simulink model "FlightGearIntegration"  (R2022b)
settings: Solver=VariableStepAuto  StartTime=0.0  StopTime=5  RelTol=1e-3
undefined symbols (not defined in the file): Pitch, Roll, Thrust, YawRate
libraries: aerolibfltsims x1, uavalgslib x1, aerolibanimutils x1
settings Model: Creator=skjet  LastModifiedBy=skjet
settings OptimizationCC: BlockReduction=off  DefaultParameterBehavior=Inlined  BufferReuse=off

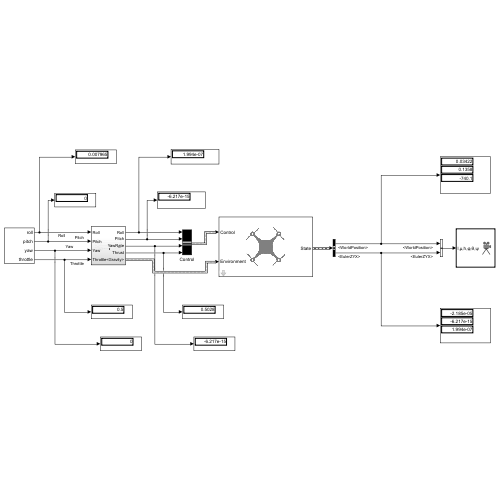
[thumbnail: Simulink's stored preview of the top-level diagram]
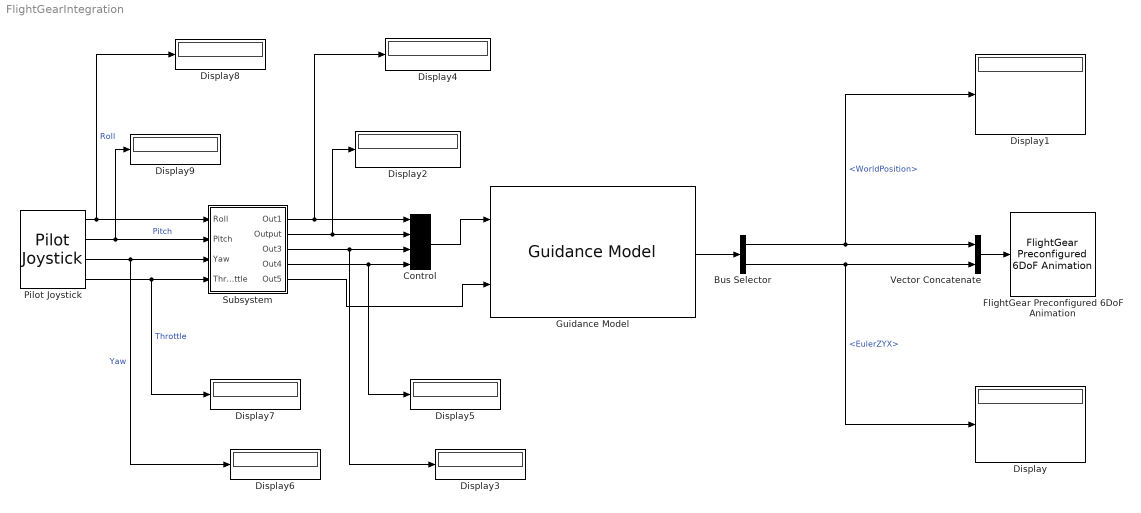
== system FlightGearIntegration ==
  Bus Selector : BusSelector  OutputSignals=WorldPosition,EulerZYX
  Control : BusCreator  Inputs=Roll,Pitch,YawRate,Thrust  OutDataTypeStr=Bus: MultirotorGuidanceControlBus  NonVirtualBus=on
  Display{,1..9} (10 alike) : Display
  FlightGear Preconfigured 6DoF Animation : aerolibfltsims/FlightGear Preconfigured 6DoF Animation  xFlightGearVersion=v2019.1  DestinationIpAddress=127.0.0.1  DestinationPort=5502  SampleTime=1/30  packetVersion=24
  Guidance Model : uavalgslib/Guidance Model  ModelType=MultirotorGuidance  SpecifiedDataType=double  SimulateUsing=Interpreted execution  InitialWorldPositionMultirotor=[0; 0; 0]  InitialWorldVelocityMultirotor=[0; 0; 0]  InitialEulerZYXMultirotor=[0; 0; 0]  InitialBodyAngularRateRPYMultirotor=[0; 0; 0]  InitialThrustMultirotor=0  InitialNorthFixedWing=0  InitialEastFixedWing=0  InitialHeightFixedWing=0  InitialAirSpeedFixedWing=0  InitialHeadingAngleFixedWing=0  InitialFlightPathAngleFixedWing=0  InitialRollAngleFixedWing=0  InitialRollAngleRateFixedWing=0  PDRollMultirotor=[3402.97,116.67]  PDPitchMultirotor=[3402.97, 116.67]  PYawRateMultirotor=1950  PThrustMultirotor=3900  MassMultirotor=0.1  PHeightFixedWing=3.9  PHeadingAngleFixedWing=3.9  PFlightPathAngleFixedWing=39  PDRollFixedWing=[3402.97, 116.67]  PAirSpeedFixedWing=1  FlightPathAngleLimitsFixedWing=[-pi/2, pi/2]  StateBusName='MultirotorGuidanceStateBus'  ControlBusName='MultirotorGuidanceControlBus'  EnvironmentBusName='MultirotorGuidanceEnvironmentBus'  DataType=double
  Pilot Joystick : aerolibanimutils/Pilot Joystick  JoystickID=Joystick1  OutputConfiguration=FourAxis  SampleTime=1/30
  Subsystem : Subsystem
  Vector Concatenate : Concatenate
  wires:
  Pilot Joystick/1 -> Display8/1, Subsystem/1(Roll)  "Roll"
  Pilot Joystick/2 -> Display9/1, Subsystem/2(Pitch)  "Pitch"
  Pilot Joystick/3 -> Display6/1, Subsystem/3(Yaw)  "Yaw"
  Pilot Joystick/4 -> Display7/1, Subsystem/4(Throttle)  "Throttle"
  Guidance Model/1 -> Bus Selector/1
  Bus Selector/1 -> Display1/1, Vector Concatenate/1  "<WorldPosition>"
  Bus Selector/2 -> Display/1, Vector Concatenate/2  "<EulerZYX>"
  Vector Concatenate/1 -> FlightGear Preconfigured 6DoF Animation/1
  Subsystem/5(Out5) -> Guidance Model/2
  Control/1 -> Guidance Model/1
  Subsystem/4(Out4) -> Display5/1, Control/4
  Subsystem/3(Out3) -> Control/3, Display3/1
  Subsystem/2(Output) -> Display2/1, Control/2
  Subsystem/1(Out1) -> Display4/1, Control/1

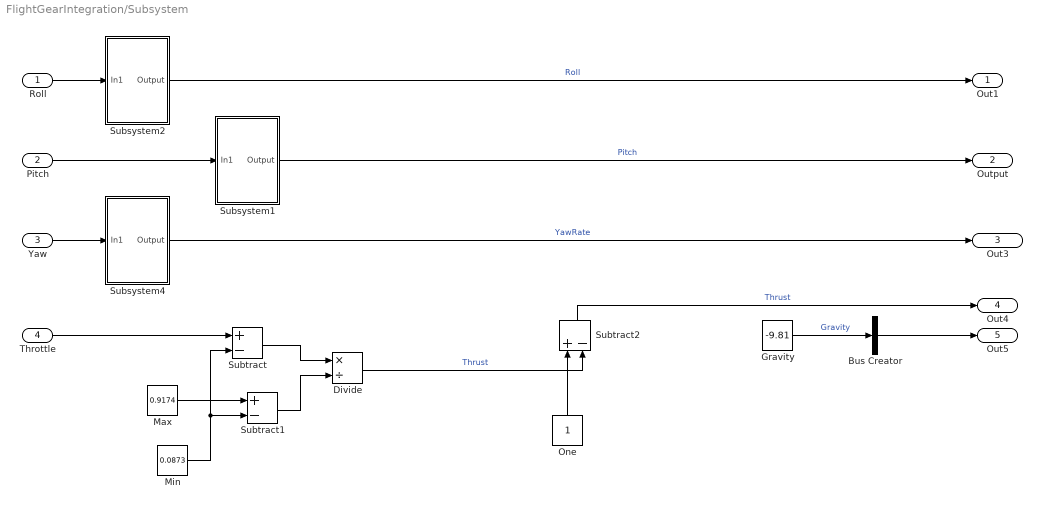
== system FlightGearIntegration/Subsystem ==
  Roll : Inport
  Pitch : Inport  Port=2
  Yaw : Inport  Port=3
  Throttle : Inport  Port=4
  Bus Creator : BusCreator  Inputs=Gravity  OutDataTypeStr=Bus: MultirotorGuidanceEnvironmentBus  NonVirtualBus=on
  Divide : Product  Inputs=*/
  Gravity : Constant  Value=-9.81
  Max : Constant  Value=0.9174
  Min : Constant  Value=0.0873
  One : Constant  OutDataTypeStr=Inherit: Inherit via back propagation
  Subsystem1 : Subsystem
  Subsystem2 : Subsystem
  Subsystem4 : Subsystem
  Subtract : Sum  Inputs=+-
  Subtract1 : Sum  Inputs=+-
  Subtract2 : Sum  Inputs=+-
  Out1 : Outport
  Output : Outport  Port=2
  Out3 : Outport  Port=3
  Out4 : Outport  Port=4
  Out5 : Outport  Port=5
  wires:
  Gravity/1 -> Bus Creator/1  "Gravity"
  Subsystem2/1(Output) -> Out1/1  "Roll"
  Subsystem4/1(Output) -> Out3/1  "YawRate"
  Bus Creator/1 -> Out5/1
  Subsystem1/1(Output) -> Output/1  "Pitch"
  Roll/1 -> Subsystem2/1(In1)
  Yaw/1 -> Subsystem4/1(In1)
  Pitch/1 -> Subsystem1/1(In1)
  Subtract1/1 -> Divide/2
  Min/1 -> Subtract/2, Subtract1/2
  Max/1 -> Subtract1/1
  Subtract/1 -> Divide/1
  Throttle/1 -> Subtract/1
  Divide/1 -> Subtract2/2  "Thrust"
  One/1 -> Subtract2/1
  Subtract2/1 -> Out4/1  "Thrust"

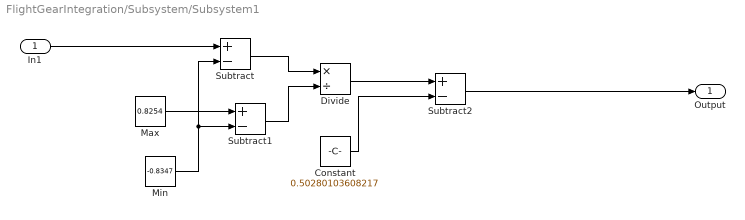
== system FlightGearIntegration/Subsystem/Subsystem1 ==
  In1 : Inport
  Constant : Constant  Value=0.50280103608217
  Divide : Product  Inputs=*/
  Max : Constant  Value=0.8254
  Min : Constant  Value=-0.8347
  Subtract : Sum  Inputs=+-
  Subtract1 : Sum  Inputs=+-
  Subtract2 : Sum  Inputs=+-
  Output : Outport
  wires:
  Divide/1 -> Subtract2/1
  Max/1 -> Subtract1/1
  In1/1 -> Subtract/1
  Min/1 -> Subtract/2, Subtract1/2
  Subtract/1 -> Divide/1
  Subtract1/1 -> Divide/2
  Subtract2/1 -> Output/1
  Constant/1 -> Subtract2/2

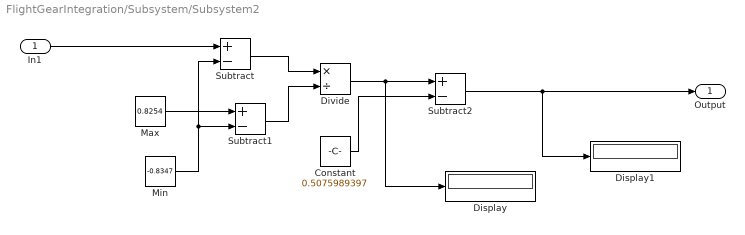
== system FlightGearIntegration/Subsystem/Subsystem2 ==
  In1 : Inport
  Constant : Constant  Value=0.5075989397
  Display : Display
  Display1 : Display
  Divide : Product  Inputs=*/
  Max : Constant  Value=0.8254
  Min : Constant  Value=-0.8347
  Subtract : Sum  Inputs=+-
  Subtract1 : Sum  Inputs=+-
  Subtract2 : Sum  Inputs=+-
  Output : Outport
  wires:
  Divide/1 -> Display/1, Subtract2/1
  Max/1 -> Subtract1/1
  In1/1 -> Subtract/1
  Min/1 -> Subtract/2, Subtract1/2
  Subtract/1 -> Divide/1
  Subtract1/1 -> Divide/2
  Subtract2/1 -> Display1/1, Output/1
  Constant/1 -> Subtract2/2

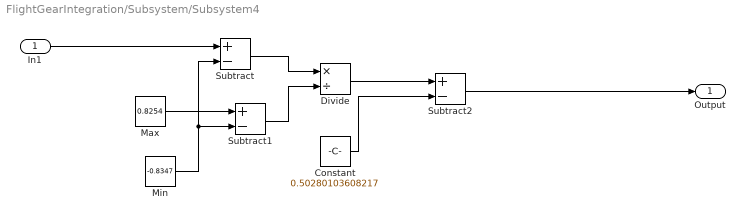
== system FlightGearIntegration/Subsystem/Subsystem4 ==
  In1 : Inport
  Constant : Constant  Value=0.50280103608217
  Divide : Product  Inputs=*/
  Max : Constant  Value=0.8254
  Min : Constant  Value=-0.8347
  Subtract : Sum  Inputs=+-
  Subtract1 : Sum  Inputs=+-
  Subtract2 : Sum  Inputs=+-
  Output : Outport
  wires:
  Divide/1 -> Subtract2/1
  Max/1 -> Subtract1/1
  In1/1 -> Subtract/1
  Min/1 -> Subtract/2, Subtract1/2
  Subtract/1 -> Divide/1
  Subtract1/1 -> Divide/2
  Subtract2/1 -> Output/1
  Constant/1 -> Subtract2/2
